simulink model "PANCslc_max"  (R2020a)
settings: Solver=ode3  StartTime=0.0  StopTime=10.0  FixedStep=0.1  RelTol=1e-3  EnableMultiTasking=on
settings Model: Creator=CARVALHO  LastModifiedBy=Arnaldo
settings DataIOCC: LimitDataPoints=on  SaveFormat=Array  ReturnWorkspaceOutputs=off
settings OptimizationCC: LifeSpan=inf
settings DebuggingCC: SFUnexpectedBacktrackingDiag=warning  SFNoUnconditionalDefaultTransitionDiag=warning  SFExecutionAtInitializationDiag=none  ArithmeticOperatorsInVariantConditions=warning
settings HardwareCC: ProdBitPerPointer=32  ProdBitPerSizeT=32  ProdBitPerPtrDiffT=32  ProdLargestAtomicFloat=None  ProdIntDivRoundTo=Undefined  ProdEndianess=Unspecified  ProdWordSize=32  ProdHWDeviceType=32-bit Generic
settings ModelReferenceCC: PropagateSignalLabelsOutOfModel=off
settings SFSimCC: SimUseLocalCustomCode=off  CustomCodeUndefinedFunction=UseInterfaceOnly
settings RTWCC: RTWUseLocalCustomCode=off
settings CodeAppCC: StateflowObjectComments=on
settings GRTTargetCC: TargetLangStandard=C89/C90 (ANSI)
settings ConfigComp: CovMetricSettings=dw  CovHtmlReporting=on  CovSaveCumulativeToWorkspaceVar=on  CovSaveSingleToWorkspaceVar=on  CovExternalEMLEnable=off

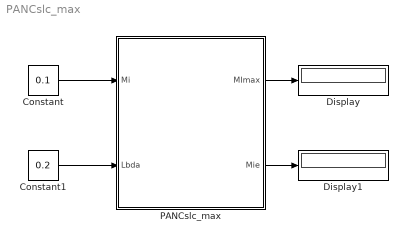
== system PANCslc_max ==
  Constant : Constant  Value=0.1
  Constant1 : Constant  Value=0.2
  Display : Display
  Display1 : Display
  PANCslc_max : Subsystem  Tag=NAP  Description=Célula de Aprendizagem NAP
  wires:
  Constant/1 -> PANCslc_max/1(Mi)
  Constant1/1 -> PANCslc_max/2(Lbda)
  PANCslc_max/1(MImax) -> Display/1
  PANCslc_max/2(Mie) -> Display1/1

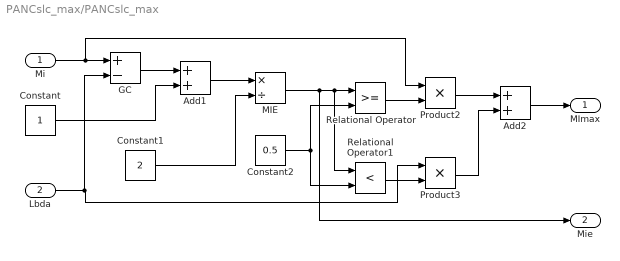
== system PANCslc_max/PANCslc_max ==
  Mi : Inport
  Lbda : Inport  Port=2
  Add1 : Sum
  Add2 : Sum
  Constant : Constant
  Constant1 : Constant  Value=2
  Constant2 : Constant  Value=0.5
  GC : Sum  Inputs=+-
  MIE : Product  Inputs=*/
  Product2 : Product  RndMeth=Zero
  Product3 : Product  RndMeth=Zero
  Relational Operator : RelationalOperator  OutDataTypeStr=boolean  RndMeth=Nearest
  Relational Operator1 : RelationalOperator  Operator=<  OutDataTypeStr=boolean  RndMeth=Nearest
  MImax : Outport
  Mie : Outport  Port=2
  wires:
  Constant/1 -> Add1/2
  Mi/1 -> Product2/1, GC/1
  GC/1 -> Add1/1
  Add1/1 -> MIE/1
  Constant1/1 -> MIE/2
  MIE/1 -> Mie/1, Relational Operator1/1, Relational Operator/1
  Constant2/1 -> Relational Operator1/2, Relational Operator/2
  Relational Operator/1 -> Product2/2
  Relational Operator1/1 -> Product3/2
  Product2/1 -> Add2/1
  Product3/1 -> Add2/2
  Add2/1 -> MImax/1
  Lbda/1 -> Product3/1, GC/2
